simulink model "model_bros_mattia"  (R2016b)
settings: Solver=FixedStepDiscrete  StartTime=0.0  StopTime=inf  FixedStep=sampleTime  RelTol=1e-3
PostLoadFcn:
  | % load model parameters
  | parameters_model_bros;
  | 
  | % set requested state
  | set_param('model_bros_mattia/Requested state','Value',num2str(0));
InitFcn:
  | % load model parameters
  | parameters_model_bros;
  | 
  | % set requested state
  | set_param('model_bros_mattia/Requested state','Value',num2str(0));
StartFcn:
  | % load model parameters
  | parameters_model_bros;
  | 
  | % set requested state
  | set_param('model_bros_mattia/Requested state','Value',num2str(0));
values from neighbouring files (symbols this model uses):
  Lb = 0.07    [parameters_model_bros.m]
  Lf = 0.238    [parameters_model_bros.m]
  Lu = 0.153    [parameters_model_bros.m]
  maxofx_target = maxofx    [parameters_model_bros.m]
  maxofy_target = maxofy    [parameters_model_bros.m]
  nx_target = nx    [parameters_model_bros.m]
  ny_target = ny    [parameters_model_bros.m]
  phasesx_target = phasesx    [parameters_model_bros.m]
  phasesy_target = phasesy    [parameters_model_bros.m]
  sampleTime = 0.001    [parameters_model_bros.m]
undefined symbols (not defined in the file or in its folder): FM1, FM2
libraries: simulink x22, LibraryFM x14, VariousBlocksLibrary x7, simulink_extras x1
(part 3 of 3)

== matlab function model_bros_mattia/Robot1/DataFromEtherCAT/FTSensor_K6D27/SensorToOperationalSpace ==
  data: q_all input; Fs input; FTOpSpace output; transmatside input
function FTOpSpace = ForceSensorToOperationalSpace(q_all,Fs,transmatside)
%#codegen
q1 = q_all(1);
q2 = q_all(2);
q4 = q_all(4);
q5 = q_all(5);

% based on which arm the force sensor is connected
switch transmatside
    case 1
        alpha = pi-q2;   
        beta = q1+alpha-pi/2;
        R0 = rotmat(beta);
        R = blkdiag(R0,R0); % transform forces and moments
    case 2
        alpha = -(pi - q4);
        beta = q5+alpha-pi/2;
        R0 = rotmat(beta);
        R = blkdiag(R0,R0); % transform forces and moments
    otherwise
        R = eye(length(Fs));
end

% transform force
FTOpSpace = R*Fs;

function R = rotmat(q)

R = [cos(q) -sin(q) 0;...
      sin(q)  cos(q) 0;...
      0       0      1];

== matlab function model_bros_mattia/Robot1/DataToEtherCAT/WorkspacePositionGuard/CheckInternalAngles ==
  data: theta input; angleError output
function angleError = checkInternalErrors(theta)
%#codegen


angleError = 0;
if any(theta([2 4]) >= 0.95*pi)
    angleError = 1;
end

== matlab function model_bros_mattia/Robot1/DataToEtherCAT/WorkspacePositionGuard/EndpointPositionGuard ==
  data: correctState input; xe input; error output
function error = fcn(correctState, xe)
%#codegen


error = 0;

% only check workspace boundaries after homing state is done
if ~correctState 
    return; 
end

% x0 = 0;
% y0 = 0.2354;
% a = 0.11;
% b = 0.08;

% workspace (see design document)
x0 = 0;
y0 = 0.25024;
a = 0.1746;
b = 0.13;%0.1048;

% check if endpoint is outside a predefined ellipse
x = xe(1);
y = xe(2);

% workspace is defined as an ellipse
e = (x-x0)^2 / a^2 + (y-y0)^2 / b^2;

% if is larger than 1, the endpoint is outside the workspace
if e > 1
    error = 1;
end
